simulink model "FirstCode_InHardware_CAN_Enable"  (R2014b)
settings: configuration reference "Embedded_Configuration" (kept outside this file)
PreLoadFcn:
  | load('Embedded_Config.mat')
PostLoadFcn:
  | c2000demoscallback(1)
model workspace: external: MAT-File Embedded_Config.mat (data not in the file)
undefined symbols (not defined in the file or in its folder): canChannel
libraries: canmsglib x2, canlib x2, c280xlib x1
settings Model: Creator=The MathWorks Inc.  LastModifiedBy=Nathan

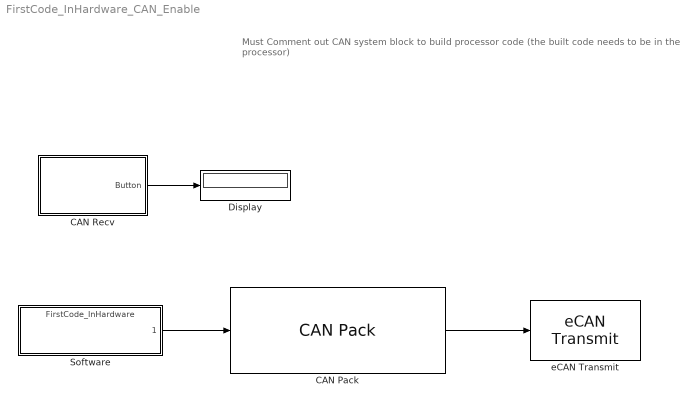
== system FirstCode_InHardware_CAN_Enable ==
  note: Must Comment out CAN system block
      | to build processor code
      | (the built code needs to be in the processor)
  CAN Pack : canmsglib/CAN Pack  MsgList=(none)  MsgName=Button  MsgIDType=Standard (11-bit identifier)  MsgIdentifier=2  MsgLength=2  SignalInfo=Button$0$16$1$1$1$0$1$0$-Inf$Inf$#  NSignals=1  StartBits=str2num('[int32(0)]')  SignalSizes=str2num('[int32(16)]')  ByteOrders=str2num('[int32(1)]')  DataTypes=str2num('[int32(1)]')  MultiplexTypes=str2num('[int32(1)]')  MultiplexValues=str2num('[double(0)]')  Factors=str2num('[double(1)]')  Offsets=str2num('[double(0)]')  Minimums=str2num('[double(-Inf)]')  Maximums=str2num('[double(Inf)]')  Remote=off
      settings: DataFormat=manually specified signals
  CAN Recv : Subsystem
  Display : Display
  Software : ModelReference  ModelNameDialog=FirstCode_InHardware.slx  SimulationMode=Normal  ModelReferenceVersion=1.90  CopyOfModelName=FirstCode_InHardware.slx  DefaultDataLogging=on
  eCAN Transmit : c280xlib/eCAN Transmit  chipFamily=C280x  useModule=eCAN_A  mailboxNo=1  messageID=2  messageType=Standard (11-bit identifier)  enableBlockingMode=off  postInterrupt=off  interruptLine=0
  wires:
  Software/1 -> CAN Pack/1
  CAN Pack/1 -> eCAN Transmit/1
  CAN Recv/1(Button) -> Display/1

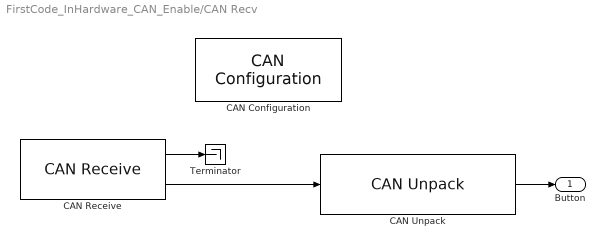
== system FirstCode_InHardware_CAN_Enable/CAN Recv ==
  CAN Configuration : canlib/CAN Configuration  BlockHandle=266.0009  DeviceMenu=Kvaser Eagle 1 (Channel 1)  Device=Kvaser Eagle 1 (Channel 1)  ObjConstructor=canChannel('Kvaser', 'Eagle 1', 1)  BusSpeed=500000  EnableBitParameters=off  SJW=1  TSEG1=4  TSEG2=3  NSamples=1  AckMode=Normal
  CAN Receive : canlib/CAN Receive  BlockHandle=246.0004  DeviceMenu=Kvaser Eagle 1 (Channel 1)  Device=Kvaser Eagle 1 (Channel 1)  ObjConstructor=canChannel('Kvaser', 'Eagle 1', 1)  EnableStandardIDsFilter=off  StandardIDs=2  EnableExtendedIDsFilter=off  ExtendedIDs=0  SampleTime=.01  MsgsPerTimestep=all  StdIDsCombo=Allow only  ExtIDsCombo=Block all  InternalFilterUpdateStatus=on
  CAN Unpack : canmsglib/CAN Unpack  MsgList=(none)  MsgName=Button  MsgIDType=Standard (11-bit identifier)  MsgIdentifier=2  MsgLength=2  SignalInfo=Button$0$16$1$1$1$0$1$0$-Inf$Inf$#  NSignals=1  IDPort=off  TimestampPort=off  ErrorPort=off  RemotePort=off  LengthPort=off  StatusPort=off  StartBits=str2num('[int32(0)]')  SignalSizes=str2num('[int32(16)]')  ByteOrders=str2num('[int32(1)]')  DataTypes=str2num('[int32(1)]')  MultiplexTypes=str2num('[int32(1)]')  MultiplexValues=str2num('[double(0)]')  Factors=str2num('[double(1)]')  Offsets=str2num('[double(0)]')  Minimums=str2num('[double(-Inf)]')  Maximums=str2num('[double(Inf)]')
  Terminator : Terminator
  Button : Outport
  wires:
  CAN Unpack/1 -> Button/1
  CAN Receive/2 -> CAN Unpack/1
  CAN Receive/1 -> Terminator/1
